simulink model "test_bu01_2018b"  (R2018b)
settings: Solver=FixedStepAuto  StartTime=0.0  StopTime=10  FixedStep=0.02  RelTol=1e-3
model workspace (MAT data in the model file):
  Ixx = 0.8
  Iyy = 2.075
  Izz = 1.25
  K = 0.75
  Mass = 11.5
  b = 0
libraries: simulink x10, aerolibutil x6, vrlib x4, sharedtransform x4, sharedutil x3, shared6dof x1
(part 2 of 4)

== system test_bu01_2018b/bu01_model/动力系统模型/Motor4_TM_N/TMU5KV400  ==
  Um : Inport  PortDimensions=1
  Tq : Inport  Port=2  PortDimensions=1
  Izz : Inport  Port=3  PortDimensions=1
  Bus Selector : BusSelector  OutputSignals=Im,RPM
  Bus Creator : BusCreator  Inputs=3
  DCMotor : Subsystem  mask{L=0.0053, Km=0.024, Kemf=0.024, Imzz=0.00002, Ra=0.113, I0=0.725}
      mask prompts: L "电感值L"; Km "转矩常量Km"; Kemf "反电动势Kemf"; Imzz "转子惯量Imzz"; Ra "电动机内阻Ra"; I0 "空载电流I0"
      mask Display: disp('DCMotor')
  Im : Outport
  RPM : Outport  Port=2
  wires:
  Bus Selector/2 -> RPM/1  "<RPM>"
  Bus Selector/1 -> Im/1  "<Im>"
  DCMotor/1(Out1) -> Bus Selector/1
  Um/1 -> Bus Creator/1  "Um"
  Bus Creator/1 -> DCMotor/1(In1)
  Izz/1 -> Bus Creator/3  "Izz"
  Tq/1 -> Bus Creator/2  "Tq"

== system test_bu01_2018b/bu01_model/动力系统模型/Motor5_PF_N/PF70mmDuctFanN ==
  Vb_ip : Inport  PortDimensions=3
  Wb_ip : Inport  Port=2  PortDimensions=3
  Ax_ip : Inport  Port=3  PortDimensions=3
  Ns_ip : Inport  Port=4  PortDimensions=1
  Pro : Inport  Port=5  PortDimensions=1
  Bus Selector : BusSelector  OutputSignals=Fb&Mb,Tq,Izz
  Bus Selector1 : BusSelector  OutputSignals=Fb,Mb
  Bus Creator : BusCreator  Inputs=5
  "涵道风扇模型 " : Subsystem  mask{Fratio=1.125, Mratio=0.975, Tqratio=0.4, Izz=0.00000309}
      mask prompts: Fratio "涵道风扇气动力修正系数"; Mratio "涵道风扇气动力矩修正系数"; Tqratio "涵道风扇扭矩修正系数"; Izz "涵道风扇转动惯量"
  Fb : Outport
  Mb : Outport  Port=2
  Tq : Outport  Port=3
  Izz : Outport  Port=4
  wires:
  Pro/1 -> Bus Creator/5  "Pro"
  Bus Selector/2 -> Tq/1  "<Tq>"
  Bus Selector/3 -> Izz/1  "<Izz>"
  Bus Selector1/1 -> Fb/1  "<Fb>"
  Ns_ip/1 -> Bus Creator/4  "Ns"
  Bus Selector1/2 -> Mb/1  "<Mb>"
  Bus Selector/1 -> Bus Selector1/1  "<Fb&Mb>"
  Wb_ip/1 -> Bus Creator/2  "Wb"
  Bus Creator/1 -> "涵道风扇模型 "/1(In1)
  "涵道风扇模型 "/1(Out1) -> Bus Selector/1
  Ax_ip/1 -> Bus Creator/3  "Ax"
  Vb_ip/1 -> Bus Creator/1  "Vb"

== system test_bu01_2018b/bu01_model/动力系统模型/Motor5_PF_N/PFKV2300 ==
  Um : Inport  PortDimensions=1
  Tq : Inport  Port=2  PortDimensions=1
  Izz : Inport  Port=3  PortDimensions=1
  Bus Selector : BusSelector  OutputSignals=Im,RPM
  Bus Creator : BusCreator  Inputs=3
  DCMotor : Subsystem  mask{L=0.0053, Km=0.0041, Kemf=0.0041, Imzz=1e-05, Ra=0.045, I0=2.35}
      mask prompts: L "电感值L"; Km "转矩常量Km"; Kemf "反电动势Kemf"; Imzz "转子惯量Imzz"; Ra "电动机内阻Ra"; I0 "空载电流I0"
      mask Display: disp('DCMotor')
  Im : Outport
  RPM : Outport  Port=2
  wires:
  Bus Creator/1 -> DCMotor/1(In1)
  Um/1 -> Bus Creator/1  "Um"
  Izz/1 -> Bus Creator/3  "Izz"
  Bus Selector/2 -> RPM/1  "<RPM>"
  Tq/1 -> Bus Creator/2  "Tq"
  DCMotor/1(Out1) -> Bus Selector/1
  Bus Selector/1 -> Im/1  "<Im>"

== system test_bu01_2018b/bu01_model/动力系统模型/Motor6_PF_N/PF70mmDuctFanN ==
  Vb_ip : Inport  PortDimensions=3
  Wb_ip : Inport  Port=2  PortDimensions=3
  Ax_ip : Inport  Port=3  PortDimensions=3
  Ns_ip : Inport  Port=4  PortDimensions=1
  Pro : Inport  Port=5  PortDimensions=1
  Bus Selector : BusSelector  OutputSignals=Fb&Mb,Tq,Izz
  Bus Selector1 : BusSelector  OutputSignals=Fb,Mb
  Bus Creator : BusCreator  Inputs=5
  "涵道风扇模型 " : Subsystem  mask{Fratio=1.125, Mratio=0.975, Tqratio=0.4, Izz=0.00000309}
      mask prompts: Fratio "涵道风扇气动力修正系数"; Mratio "涵道风扇气动力矩修正系数"; Tqratio "涵道风扇扭矩修正系数"; Izz "涵道风扇转动惯量"
  Fb : Outport
  Mb : Outport  Port=2
  Tq : Outport  Port=3
  Izz : Outport  Port=4
  wires:
  Pro/1 -> Bus Creator/5  "Pro"
  Bus Selector/2 -> Tq/1  "<Tq>"
  Bus Selector/3 -> Izz/1  "<Izz>"
  Bus Selector1/1 -> Fb/1  "<Fb>"
  Ns_ip/1 -> Bus Creator/4  "Ns"
  Bus Selector1/2 -> Mb/1  "<Mb>"
  Bus Selector/1 -> Bus Selector1/1  "<Fb&Mb>"
  Wb_ip/1 -> Bus Creator/2  "Wb"
  Bus Creator/1 -> "涵道风扇模型 "/1(In1)
  "涵道风扇模型 "/1(Out1) -> Bus Selector/1
  Ax_ip/1 -> Bus Creator/3  "Ax"
  Vb_ip/1 -> Bus Creator/1  "Vb"

== system test_bu01_2018b/bu01_model/动力系统模型/Motor6_PF_N/PFKV2300 ==
  Um : Inport  PortDimensions=1
  Tq : Inport  Port=2  PortDimensions=1
  Izz : Inport  Port=3  PortDimensions=1
  Bus Selector : BusSelector  OutputSignals=Im,RPM
  Bus Creator : BusCreator  Inputs=3
  DCMotor : Subsystem  mask{L=0.0053, Km=0.0041, Kemf=0.0041, Imzz=1e-05, Ra=0.045, I0=2.35}
      mask prompts: L "电感值L"; Km "转矩常量Km"; Kemf "反电动势Kemf"; Imzz "转子惯量Imzz"; Ra "电动机内阻Ra"; I0 "空载电流I0"
      mask Display: disp('DCMotor')
  Im : Outport
  RPM : Outport  Port=2
  wires:
  Bus Creator/1 -> DCMotor/1(In1)
  Um/1 -> Bus Creator/1  "Um"
  Izz/1 -> Bus Creator/3  "Izz"
  Bus Selector/2 -> RPM/1  "<RPM>"
  Tq/1 -> Bus Creator/2  "Tq"
  DCMotor/1(Out1) -> Bus Selector/1
  Bus Selector/1 -> Im/1  "<Im>"

== system test_bu01_2018b/bu01_model/动力系统模型/Motor7_PF_N/PF70mmDuctFanN ==
  Vb_ip : Inport  PortDimensions=3
  Wb_ip : Inport  Port=2  PortDimensions=3
  Ax_ip : Inport  Port=3  PortDimensions=3
  Ns_ip : Inport  Port=4  PortDimensions=1
  Pro : Inport  Port=5  PortDimensions=1
  Bus Selector : BusSelector  OutputSignals=Fb&Mb,Tq,Izz
  Bus Selector1 : BusSelector  OutputSignals=Fb,Mb
  Bus Creator : BusCreator  Inputs=5
  "涵道风扇模型 " : Subsystem  mask{Fratio=1.125, Mratio=0.975, Tqratio=0.4, Izz=0.00000309}
      mask prompts: Fratio "涵道风扇气动力修正系数"; Mratio "涵道风扇气动力矩修正系数"; Tqratio "涵道风扇扭矩修正系数"; Izz "涵道风扇转动惯量"
  Fb : Outport
  Mb : Outport  Port=2
  Tq : Outport  Port=3
  Izz : Outport  Port=4
  wires:
  Pro/1 -> Bus Creator/5  "Pro"
  Bus Selector/2 -> Tq/1  "<Tq>"
  Bus Selector/3 -> Izz/1  "<Izz>"
  Bus Selector1/1 -> Fb/1  "<Fb>"
  Ns_ip/1 -> Bus Creator/4  "Ns"
  Bus Selector1/2 -> Mb/1  "<Mb>"
  Bus Selector/1 -> Bus Selector1/1  "<Fb&Mb>"
  Wb_ip/1 -> Bus Creator/2  "Wb"
  Bus Creator/1 -> "涵道风扇模型 "/1(In1)
  "涵道风扇模型 "/1(Out1) -> Bus Selector/1
  Ax_ip/1 -> Bus Creator/3  "Ax"
  Vb_ip/1 -> Bus Creator/1  "Vb"

== system test_bu01_2018b/bu01_model/动力系统模型/Motor7_PF_N/PFKV2300 ==
  Um : Inport  PortDimensions=1
  Tq : Inport  Port=2  PortDimensions=1
  Izz : Inport  Port=3  PortDimensions=1
  Bus Selector : BusSelector  OutputSignals=Im,RPM
  Bus Creator : BusCreator  Inputs=3
  DCMotor : Subsystem  mask{L=0.0053, Km=0.0041, Kemf=0.0041, Imzz=1e-05, Ra=0.045, I0=2.35}
      mask prompts: L "电感值L"; Km "转矩常量Km"; Kemf "反电动势Kemf"; Imzz "转子惯量Imzz"; Ra "电动机内阻Ra"; I0 "空载电流I0"
      mask Display: disp('DCMotor')
  Im : Outport
  RPM : Outport  Port=2
  wires:
  Bus Creator/1 -> DCMotor/1(In1)
  Um/1 -> Bus Creator/1  "Um"
  Izz/1 -> Bus Creator/3  "Izz"
  Bus Selector/2 -> RPM/1  "<RPM>"
  Tq/1 -> Bus Creator/2  "Tq"
  DCMotor/1(Out1) -> Bus Selector/1
  Bus Selector/1 -> Im/1  "<Im>"

== system test_bu01_2018b/bu01_model/动力系统模型/Motor8_PF_N/PF70mmDuctFanN ==
  Vb_ip : Inport  PortDimensions=3
  Wb_ip : Inport  Port=2  PortDimensions=3
  Ax_ip : Inport  Port=3  PortDimensions=3
  Ns_ip : Inport  Port=4  PortDimensions=1
  Pro : Inport  Port=5  PortDimensions=1
  Bus Selector : BusSelector  OutputSignals=Fb&Mb,Tq,Izz
  Bus Selector1 : BusSelector  OutputSignals=Fb,Mb
  Bus Creator : BusCreator  Inputs=5
  "涵道风扇模型 " : Subsystem  mask{Fratio=1.125, Mratio=0.975, Tqratio=0.4, Izz=0.00000309}
      mask prompts: Fratio "涵道风扇气动力修正系数"; Mratio "涵道风扇气动力矩修正系数"; Tqratio "涵道风扇扭矩修正系数"; Izz "涵道风扇转动惯量"
  Fb : Outport
  Mb : Outport  Port=2
  Tq : Outport  Port=3
  Izz : Outport  Port=4
  wires:
  Vb_ip/1 -> Bus Creator/1  "Vb"
  Ax_ip/1 -> Bus Creator/3  "Ax"
  "涵道风扇模型 "/1(Out1) -> Bus Selector/1
  Bus Creator/1 -> "涵道风扇模型 "/1(In1)
  Wb_ip/1 -> Bus Creator/2  "Wb"
  Bus Selector/1 -> Bus Selector1/1  "<Fb&Mb>"
  Bus Selector1/2 -> Mb/1  "<Mb>"
  Ns_ip/1 -> Bus Creator/4  "Ns"
  Bus Selector1/1 -> Fb/1  "<Fb>"
  Bus Selector/3 -> Izz/1  "<Izz>"
  Bus Selector/2 -> Tq/1  "<Tq>"
  Pro/1 -> Bus Creator/5  "Pro"

== system test_bu01_2018b/bu01_model/动力系统模型/Motor8_PF_N/PFKV2300 ==
  Um : Inport  PortDimensions=1
  Tq : Inport  Port=2  PortDimensions=1
  Izz : Inport  Port=3  PortDimensions=1
  Bus Selector : BusSelector  OutputSignals=Im,RPM
  Bus Creator : BusCreator  Inputs=3
  DCMotor : Subsystem  mask{L=0.0053, Km=0.0041, Kemf=0.0041, Imzz=1e-05, Ra=0.045, I0=2.35}
      mask prompts: L "电感值L"; Km "转矩常量Km"; Kemf "反电动势Kemf"; Imzz "转子惯量Imzz"; Ra "电动机内阻Ra"; I0 "空载电流I0"
      mask Display: disp('DCMotor')
  Im : Outport
  RPM : Outport  Port=2
  wires:
  Bus Selector/1 -> Im/1  "<Im>"
  DCMotor/1(Out1) -> Bus Selector/1
  Tq/1 -> Bus Creator/2  "Tq"
  Bus Selector/2 -> RPM/1  "<RPM>"
  Izz/1 -> Bus Creator/3  "Izz"
  Um/1 -> Bus Creator/1  "Um"
  Bus Creator/1 -> DCMotor/1(In1)

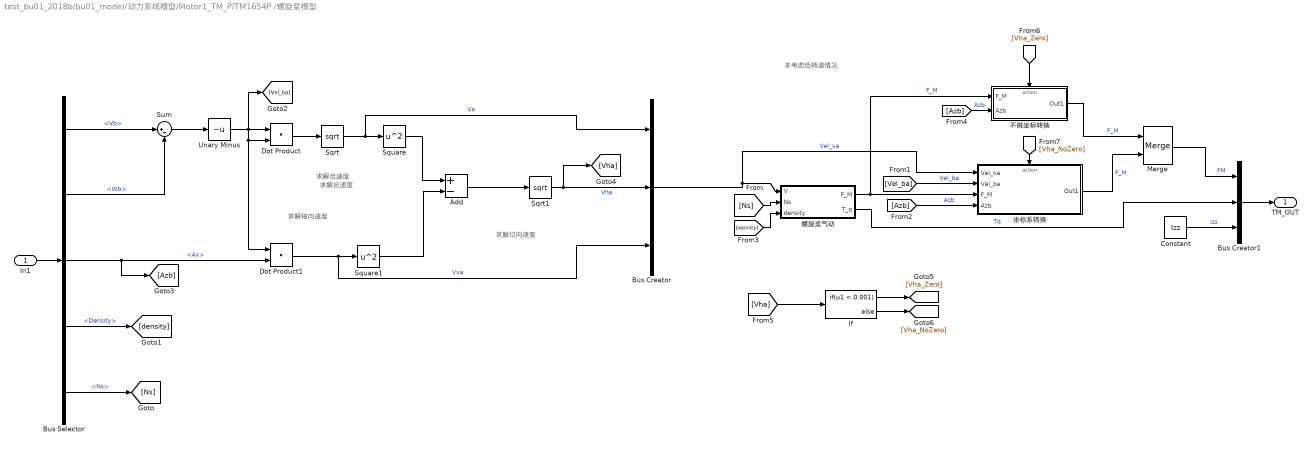
== system test_bu01_2018b/bu01_model/动力系统模型/Motor1_TM_P/TM1654P /螺旋桨模型 ==
  note: 未考虑低转速情况
  note: 求解合速度
  note: 求解轴向速度
  note: 求解切向速度
  note: 求解合速度
  In1 : Inport
  Add : Sum  Inputs=+-
  Bus Selector : BusSelector  OutputSignals=Vb,Wb,Ax,Density,Ns
  Bus Creator : BusCreator  Inputs=3
  Bus Creator1 : BusCreator  Inputs=3
  Constant : Constant  Value=Izz  OutDataTypeStr=double
  Dot Product : DotProduct  InputSameDT=on  OutDataTypeStr=Inherit: Inherit via internal rule
  Dot Product1 : DotProduct  InputSameDT=on  OutDataTypeStr=Inherit: Inherit via internal rule
  If : If  IfExpression=u1 < 0.001
  Merge : Merge
  Sqrt : Sqrt  SaturateOnIntegerOverflow=on
  Sqrt1 : Sqrt  SaturateOnIntegerOverflow=on
  Square : Math  Operator=square  SaturateOnIntegerOverflow=on
  Square1 : Math  Operator=square  SaturateOnIntegerOverflow=on
  Sum : Sum  Inputs=|+-
  Unary Minus : UnaryMinus
  不做坐标转换 : Subsystem
  坐标系转换 : Subsystem
  螺旋桨气动 : Subsystem
  TM_OUT : Outport
  wires:
  In1/1 -> Bus Selector/1
  Bus Selector/1 -> Sum/1  "<Vb>"
  Bus Selector/2 -> Sum/2  "<Wb>"
  Sum/1 -> Unary Minus/1
  Unary Minus/1 -> [Vel_ba], Dot Product/2, Dot Product1/1, Dot Product/1
  Dot Product/1 -> Sqrt/1
  Sqrt/1 -> Bus Creator/1, Square/1  "Va"
  Bus Selector/3 -> [Azb], Dot Product1/2  "<Ax>"
  Bus Selector/4 -> [density]  "<Density>"
  Bus Selector/5 -> [Ns]  "<Ns>"
  Dot Product1/1 -> Bus Creator/3, Square1/1  "Vva"
  Square1/1 -> Add/2
  Square/1 -> Add/1
  Add/1 -> Sqrt1/1
  Sqrt1/1 -> [Vha], Bus Creator/2  "Vha"
  Bus Creator/1 -> 坐标系转换/1(Vel_va), 螺旋桨气动/1(V)  "Vel_va"
  [Ns] -> 螺旋桨气动/2(Ns)
  [Vel_ba] -> 坐标系转换/2(Vel_ba)  "Vel_ba"
  螺旋桨气动/1(F_M) -> 不做坐标转换/1(F_M), 坐标系转换/3(F_M)  "F_M"
  [Azb] -> 坐标系转换/4(Azb)  "Azb"
  [density] -> 螺旋桨气动/3(density)
  螺旋桨气动/2(T_q) -> Bus Creator1/2  "Tq"
  Constant/1 -> Bus Creator1/3  "Izz"
  Bus Creator1/1 -> TM_OUT/1
  [Azb] -> 不做坐标转换/2(Azb)  "Azb"
  [Vha] -> If/1
  不做坐标转换/1(Out1) -> Merge/1  "F_M"
  坐标系转换/1(Out1) -> Merge/2  "F_M"
  Merge/1 -> Bus Creator1/1  "FM"
  If/1 -> [Vha_Zero]
  If/2 -> [Vha_NoZero]
  [Vha_Zero] -> 不做坐标转换/Action
  [Vha_NoZero] -> 坐标系转换/Action

== system test_bu01_2018b/bu01_model/动力系统模型/Motor1_TM_P/TMU5KV400 /DCMotor ==
  In1 : Inport
  Add : Sum  Inputs=+--
  Add1 : Sum  Inputs=+-
  Add2 : Sum
  Add3 : Sum  Inputs=+-
  Bus Selector : BusSelector  OutputSignals=Um,Tq,Izz
  Bus Creator : BusCreator  Inputs=2
  Constant : Constant  Value=Imzz
  Constant1 : Constant  Value=I0
  Divide : Product  Inputs=*/
  Gain : Gain  Gain=1/L
  Gain1 : Gain  Gain=Km
  Gain3 : Gain  Gain=Kemf
  Gain4 : Gain  Gain=Ra
  Gain5 : Gain  Gain=1/(2*pi)
  Gain6 : Gain  Gain=60
  Integrator : Integrator  InitialCondition=0.0001
  Integrator1 : Integrator  InitialCondition=0.0001
  Multiply : Product
  Multiply1 : Product
  Terminator : Terminator
  Terminator1 : Terminator
  Out1 : Outport
  wires:
  In1/1 -> Bus Selector/1
  Bus Selector/1 -> Multiply/1, Add/1  "<Um>"
  Add/1 -> Gain/1
  Gain/1 -> Integrator/1
  Integrator/1 -> Add3/1, Multiply/2, Bus Creator/1, Gain4/1  "Im"
  Gain1/1 -> Multiply1/1, Add1/1  "Te"
  Integrator1/1 -> Multiply1/2, Gain3/1, Gain5/1  "w"
  Add1/1 -> Divide/1
  Divide/1 -> Integrator1/1
  Gain3/1 -> Add/2  "Ea"
  Gain4/1 -> Add/3
  Bus Selector/2 -> [Tq]  "<Tq>"
  Bus Selector/3 -> Add2/1  "<Izz>"
  Constant/1 -> Add2/2
  Add2/1 -> [J]
  [J] -> Divide/2
  Multiply/1 -> Terminator/1  "Pwin"
  Multiply1/1 -> Terminator1/1  "Pwout"
  Gain5/1 -> Gain6/1  "RPS"
  Gain6/1 -> Bus Creator/2  "RPM"
  Bus Creator/1 -> Out1/1
  [Tq] -> Add1/2
  Add3/1 -> Gain1/1  "Iav"
  Constant1/1 -> Add3/2

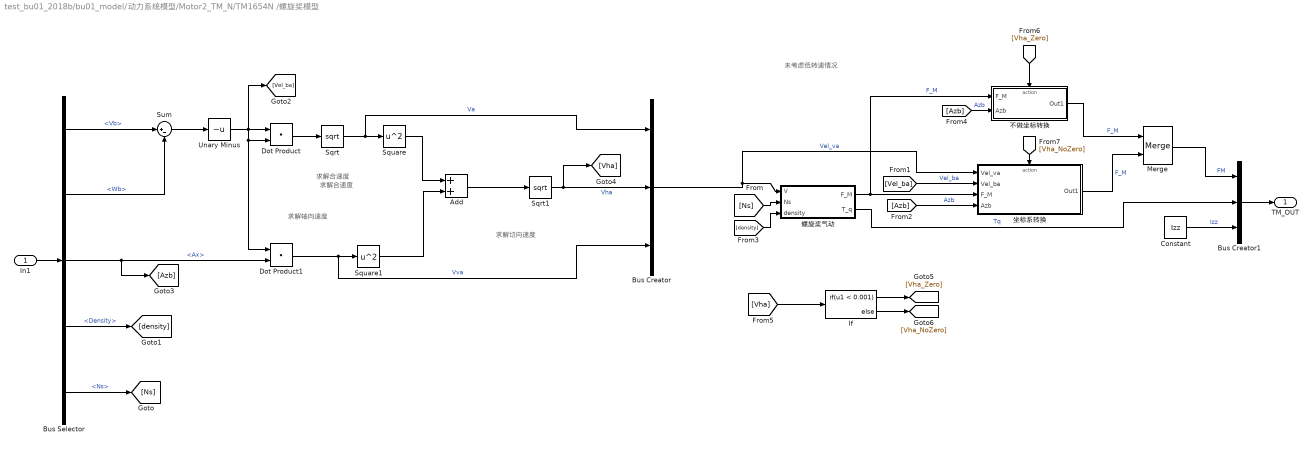
== system test_bu01_2018b/bu01_model/动力系统模型/Motor2_TM_N/TM1654N /螺旋桨模型 ==
  note: 未考虑低转速情况
  note: 求解合速度
  note: 求解轴向速度
  note: 求解切向速度
  note: 求解合速度
  In1 : Inport
  Add : Sum
  Bus Selector : BusSelector  OutputSignals=Vb,Wb,Ax,Density,Ns
  Bus Creator : BusCreator  Inputs=3
  Bus Creator1 : BusCreator  Inputs=3
  Constant : Constant  Value=Izz  OutDataTypeStr=double
  Dot Product : DotProduct  InputSameDT=on  OutDataTypeStr=Inherit: Inherit via internal rule
  Dot Product1 : DotProduct  InputSameDT=on  OutDataTypeStr=Inherit: Inherit via internal rule
  If : If  IfExpression=u1 < 0.001
  Merge : Merge
  Sqrt : Sqrt  SaturateOnIntegerOverflow=on
  Sqrt1 : Sqrt  SaturateOnIntegerOverflow=on
  Square : Math  Operator=square  SaturateOnIntegerOverflow=on
  Square1 : Math  Operator=square  SaturateOnIntegerOverflow=on
  Sum : Sum  Inputs=|+-
  Unary Minus : UnaryMinus
  不做坐标转换 : Subsystem
  坐标系转换 : Subsystem
  螺旋桨气动 : Subsystem
  TM_OUT : Outport
  wires:
  In1/1 -> Bus Selector/1
  Bus Selector/1 -> Sum/1  "<Vb>"
  Bus Selector/2 -> Sum/2  "<Wb>"
  Sum/1 -> Unary Minus/1
  Unary Minus/1 -> [Vel_ba], Dot Product/2, Dot Product1/1, Dot Product/1
  Dot Product/1 -> Sqrt/1
  Sqrt/1 -> Bus Creator/1, Square/1  "Va"
  Bus Selector/3 -> [Azb], Dot Product1/2  "<Ax>"
  Bus Selector/4 -> [density]  "<Density>"
  Bus Selector/5 -> [Ns]  "<Ns>"
  Dot Product1/1 -> Bus Creator/3, Square1/1  "Vva"
  Square1/1 -> Add/2
  Square/1 -> Add/1
  Add/1 -> Sqrt1/1
  Sqrt1/1 -> [Vha], Bus Creator/2  "Vha"
  Bus Creator/1 -> 坐标系转换/1(Vel_va), 螺旋桨气动/1(V)  "Vel_va"
  [Ns] -> 螺旋桨气动/2(Ns)
  [Vel_ba] -> 坐标系转换/2(Vel_ba)  "Vel_ba"
  螺旋桨气动/1(F_M) -> 不做坐标转换/1(F_M), 坐标系转换/3(F_M)  "F_M"
  [Azb] -> 坐标系转换/4(Azb)  "Azb"
  [density] -> 螺旋桨气动/3(density)
  螺旋桨气动/2(T_q) -> Bus Creator1/2  "Tq"
  Constant/1 -> Bus Creator1/3  "Izz"
  Bus Creator1/1 -> TM_OUT/1
  [Azb] -> 不做坐标转换/2(Azb)  "Azb"
  [Vha] -> If/1
  不做坐标转换/1(Out1) -> Merge/1  "F_M"
  坐标系转换/1(Out1) -> Merge/2  "F_M"
  Merge/1 -> Bus Creator1/1  "FM"
  If/1 -> [Vha_Zero]
  If/2 -> [Vha_NoZero]
  [Vha_Zero] -> 不做坐标转换/Action
  [Vha_NoZero] -> 坐标系转换/Action

== system test_bu01_2018b/bu01_model/动力系统模型/Motor2_TM_N/TMU5KV400 /DCMotor ==
  In1 : Inport
  Add : Sum  Inputs=+--
  Add1 : Sum  Inputs=+-
  Add2 : Sum
  Add3 : Sum  Inputs=+-
  Bus Selector : BusSelector  OutputSignals=Um,Tq,Izz
  Bus Creator : BusCreator  Inputs=2
  Constant : Constant  Value=Imzz
  Constant1 : Constant  Value=I0
  Divide : Product  Inputs=*/
  Gain : Gain  Gain=1/L
  Gain1 : Gain  Gain=Km
  Gain3 : Gain  Gain=Kemf
  Gain4 : Gain  Gain=Ra
  Gain5 : Gain  Gain=1/(2*pi)
  Gain6 : Gain  Gain=60
  Integrator : Integrator  InitialCondition=0.0001
  Integrator1 : Integrator  InitialCondition=0.0001
  Multiply : Product
  Multiply1 : Product
  Terminator : Terminator
  Terminator1 : Terminator
  Out1 : Outport
  wires:
  In1/1 -> Bus Selector/1
  Bus Selector/1 -> Multiply/1, Add/1  "<Um>"
  Add/1 -> Gain/1
  Gain/1 -> Integrator/1
  Integrator/1 -> Add3/1, Multiply/2, Bus Creator/1, Gain4/1  "Im"
  Gain1/1 -> Multiply1/1, Add1/1  "Te"
  Integrator1/1 -> Multiply1/2, Gain3/1, Gain5/1  "w"
  Add1/1 -> Divide/1
  Divide/1 -> Integrator1/1
  Gain3/1 -> Add/2  "Ea"
  Gain4/1 -> Add/3
  Bus Selector/2 -> [Tq]  "<Tq>"
  Bus Selector/3 -> Add2/1  "<Izz>"
  Constant/1 -> Add2/2
  Add2/1 -> [J]
  [J] -> Divide/2
  Multiply/1 -> Terminator/1  "Pwin"
  Multiply1/1 -> Terminator1/1  "Pwout"
  Gain5/1 -> Gain6/1  "RPS"
  Gain6/1 -> Bus Creator/2  "RPM"
  Bus Creator/1 -> Out1/1
  [Tq] -> Add1/2
  Add3/1 -> Gain1/1  "Iav"
  Constant1/1 -> Add3/2

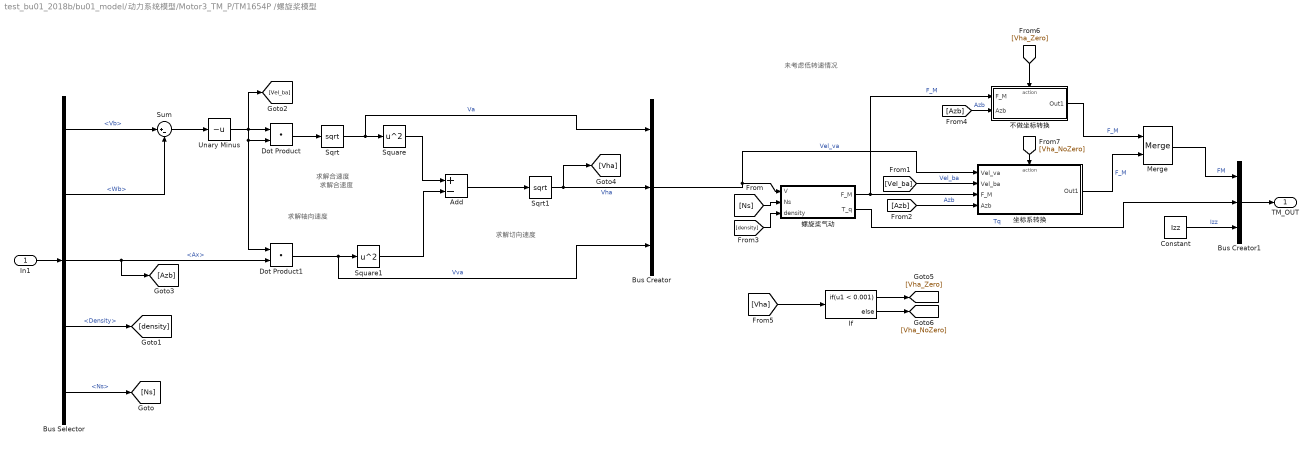
== system test_bu01_2018b/bu01_model/动力系统模型/Motor3_TM_P/TM1654P /螺旋桨模型 ==
  note: 未考虑低转速情况
  note: 求解合速度
  note: 求解轴向速度
  note: 求解切向速度
  note: 求解合速度
  In1 : Inport
  Add : Sum  Inputs=+-
  Bus Selector : BusSelector  OutputSignals=Vb,Wb,Ax,Density,Ns
  Bus Creator : BusCreator  Inputs=3
  Bus Creator1 : BusCreator  Inputs=3
  Constant : Constant  Value=Izz  OutDataTypeStr=double
  Dot Product : DotProduct  InputSameDT=on  OutDataTypeStr=Inherit: Inherit via internal rule
  Dot Product1 : DotProduct  InputSameDT=on  OutDataTypeStr=Inherit: Inherit via internal rule
  If : If  IfExpression=u1 < 0.001
  Merge : Merge
  Sqrt : Sqrt  SaturateOnIntegerOverflow=on
  Sqrt1 : Sqrt  SaturateOnIntegerOverflow=on
  Square : Math  Operator=square  SaturateOnIntegerOverflow=on
  Square1 : Math  Operator=square  SaturateOnIntegerOverflow=on
  Sum : Sum  Inputs=|+-
  Unary Minus : UnaryMinus
  不做坐标转换 : Subsystem
  坐标系转换 : Subsystem
  螺旋桨气动 : Subsystem
  TM_OUT : Outport
  wires:
  In1/1 -> Bus Selector/1
  Bus Selector/1 -> Sum/1  "<Vb>"
  Bus Selector/2 -> Sum/2  "<Wb>"
  Sum/1 -> Unary Minus/1
  Unary Minus/1 -> [Vel_ba], Dot Product/2, Dot Product1/1, Dot Product/1
  Dot Product/1 -> Sqrt/1
  Sqrt/1 -> Bus Creator/1, Square/1  "Va"
  Bus Selector/3 -> [Azb], Dot Product1/2  "<Ax>"
  Bus Selector/4 -> [density]  "<Density>"
  Bus Selector/5 -> [Ns]  "<Ns>"
  Dot Product1/1 -> Bus Creator/3, Square1/1  "Vva"
  Square1/1 -> Add/2
  Square/1 -> Add/1
  Add/1 -> Sqrt1/1
  Sqrt1/1 -> [Vha], Bus Creator/2  "Vha"
  Bus Creator/1 -> 坐标系转换/1(Vel_va), 螺旋桨气动/1(V)  "Vel_va"
  [Ns] -> 螺旋桨气动/2(Ns)
  [Vel_ba] -> 坐标系转换/2(Vel_ba)  "Vel_ba"
  螺旋桨气动/1(F_M) -> 不做坐标转换/1(F_M), 坐标系转换/3(F_M)  "F_M"
  [Azb] -> 坐标系转换/4(Azb)  "Azb"
  [density] -> 螺旋桨气动/3(density)
  螺旋桨气动/2(T_q) -> Bus Creator1/2  "Tq"
  Constant/1 -> Bus Creator1/3  "Izz"
  Bus Creator1/1 -> TM_OUT/1
  [Azb] -> 不做坐标转换/2(Azb)  "Azb"
  [Vha] -> If/1
  不做坐标转换/1(Out1) -> Merge/1  "F_M"
  坐标系转换/1(Out1) -> Merge/2  "F_M"
  Merge/1 -> Bus Creator1/1  "FM"
  If/1 -> [Vha_Zero]
  If/2 -> [Vha_NoZero]
  [Vha_Zero] -> 不做坐标转换/Action
  [Vha_NoZero] -> 坐标系转换/Action

== system test_bu01_2018b/bu01_model/动力系统模型/Motor3_TM_P/TMU5KV400 /DCMotor ==
  In1 : Inport
  Add : Sum  Inputs=+--
  Add1 : Sum  Inputs=+-
  Add2 : Sum
  Add3 : Sum  Inputs=+-
  Bus Selector : BusSelector  OutputSignals=Um,Tq,Izz
  Bus Creator : BusCreator  Inputs=2
  Constant : Constant  Value=Imzz
  Constant1 : Constant  Value=I0
  Divide : Product  Inputs=*/
  Gain : Gain  Gain=1/L
  Gain1 : Gain  Gain=Km
  Gain3 : Gain  Gain=Kemf
  Gain4 : Gain  Gain=Ra
  Gain5 : Gain  Gain=1/(2*pi)
  Gain6 : Gain  Gain=60
  Integrator : Integrator  InitialCondition=0.0001
  Integrator1 : Integrator  InitialCondition=0.0001
  Multiply : Product
  Multiply1 : Product
  Terminator : Terminator
  Terminator1 : Terminator
  Out1 : Outport
  wires:
  In1/1 -> Bus Selector/1
  Bus Selector/1 -> Multiply/1, Add/1  "<Um>"
  Add/1 -> Gain/1
  Gain/1 -> Integrator/1
  Integrator/1 -> Add3/1, Multiply/2, Bus Creator/1, Gain4/1  "Im"
  Gain1/1 -> Multiply1/1, Add1/1  "Te"
  Integrator1/1 -> Multiply1/2, Gain3/1, Gain5/1  "w"
  Add1/1 -> Divide/1
  Divide/1 -> Integrator1/1
  Gain3/1 -> Add/2  "Ea"
  Gain4/1 -> Add/3
  Bus Selector/2 -> [Tq]  "<Tq>"
  Bus Selector/3 -> Add2/1  "<Izz>"
  Constant/1 -> Add2/2
  Add2/1 -> [J]
  [J] -> Divide/2
  Multiply/1 -> Terminator/1  "Pwin"
  Multiply1/1 -> Terminator1/1  "Pwout"
  Gain5/1 -> Gain6/1  "RPS"
  Gain6/1 -> Bus Creator/2  "RPM"
  Bus Creator/1 -> Out1/1
  [Tq] -> Add1/2
  Add3/1 -> Gain1/1  "Iav"
  Constant1/1 -> Add3/2

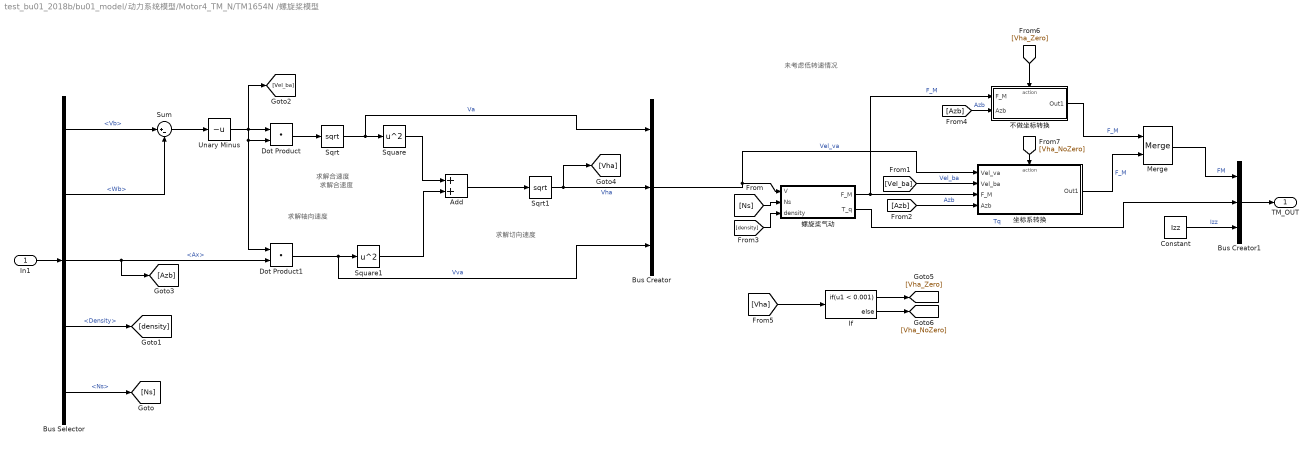
== system test_bu01_2018b/bu01_model/动力系统模型/Motor4_TM_N/TM1654N /螺旋桨模型 ==
  note: 未考虑低转速情况
  note: 求解合速度
  note: 求解轴向速度
  note: 求解切向速度
  note: 求解合速度
  In1 : Inport
  Add : Sum
  Bus Selector : BusSelector  OutputSignals=Vb,Wb,Ax,Density,Ns
  Bus Creator : BusCreator  Inputs=3
  Bus Creator1 : BusCreator  Inputs=3
  Constant : Constant  Value=Izz  OutDataTypeStr=double
  Dot Product : DotProduct  InputSameDT=on  OutDataTypeStr=Inherit: Inherit via internal rule
  Dot Product1 : DotProduct  InputSameDT=on  OutDataTypeStr=Inherit: Inherit via internal rule
  If : If  IfExpression=u1 < 0.001
  Merge : Merge
  Sqrt : Sqrt  SaturateOnIntegerOverflow=on
  Sqrt1 : Sqrt  SaturateOnIntegerOverflow=on
  Square : Math  Operator=square  SaturateOnIntegerOverflow=on
  Square1 : Math  Operator=square  SaturateOnIntegerOverflow=on
  Sum : Sum  Inputs=|+-
  Unary Minus : UnaryMinus
  不做坐标转换 : Subsystem
  坐标系转换 : Subsystem
  螺旋桨气动 : Subsystem
  TM_OUT : Outport
  wires:
  In1/1 -> Bus Selector/1
  Bus Selector/1 -> Sum/1  "<Vb>"
  Bus Selector/2 -> Sum/2  "<Wb>"
  Sum/1 -> Unary Minus/1
  Unary Minus/1 -> [Vel_ba], Dot Product/2, Dot Product1/1, Dot Product/1
  Dot Product/1 -> Sqrt/1
  Sqrt/1 -> Bus Creator/1, Square/1  "Va"
  Bus Selector/3 -> [Azb], Dot Product1/2  "<Ax>"
  Bus Selector/4 -> [density]  "<Density>"
  Bus Selector/5 -> [Ns]  "<Ns>"
  Dot Product1/1 -> Bus Creator/3, Square1/1  "Vva"
  Square1/1 -> Add/2
  Square/1 -> Add/1
  Add/1 -> Sqrt1/1
  Sqrt1/1 -> [Vha], Bus Creator/2  "Vha"
  Bus Creator/1 -> 坐标系转换/1(Vel_va), 螺旋桨气动/1(V)  "Vel_va"
  [Ns] -> 螺旋桨气动/2(Ns)
  [Vel_ba] -> 坐标系转换/2(Vel_ba)  "Vel_ba"
  螺旋桨气动/1(F_M) -> 不做坐标转换/1(F_M), 坐标系转换/3(F_M)  "F_M"
  [Azb] -> 坐标系转换/4(Azb)  "Azb"
  [density] -> 螺旋桨气动/3(density)
  螺旋桨气动/2(T_q) -> Bus Creator1/2  "Tq"
  Constant/1 -> Bus Creator1/3  "Izz"
  Bus Creator1/1 -> TM_OUT/1
  [Azb] -> 不做坐标转换/2(Azb)  "Azb"
  [Vha] -> If/1
  不做坐标转换/1(Out1) -> Merge/1  "F_M"
  坐标系转换/1(Out1) -> Merge/2  "F_M"
  Merge/1 -> Bus Creator1/1  "FM"
  If/1 -> [Vha_Zero]
  If/2 -> [Vha_NoZero]
  [Vha_Zero] -> 不做坐标转换/Action
  [Vha_NoZero] -> 坐标系转换/Action

== system test_bu01_2018b/bu01_model/动力系统模型/Motor4_TM_N/TMU5KV400 /DCMotor ==
  In1 : Inport
  Add : Sum  Inputs=+--
  Add1 : Sum  Inputs=+-
  Add2 : Sum
  Add3 : Sum  Inputs=+-
  Bus Selector : BusSelector  OutputSignals=Um,Tq,Izz
  Bus Creator : BusCreator  Inputs=2
  Constant : Constant  Value=Imzz
  Constant1 : Constant  Value=I0
  Divide : Product  Inputs=*/
  Gain : Gain  Gain=1/L
  Gain1 : Gain  Gain=Km
  Gain3 : Gain  Gain=Kemf
  Gain4 : Gain  Gain=Ra
  Gain5 : Gain  Gain=1/(2*pi)
  Gain6 : Gain  Gain=60
  Integrator : Integrator  InitialCondition=0.0001
  Integrator1 : Integrator  InitialCondition=0.0001
  Multiply : Product
  Multiply1 : Product
  Terminator : Terminator
  Terminator1 : Terminator
  Out1 : Outport
  wires:
  In1/1 -> Bus Selector/1
  Bus Selector/1 -> Multiply/1, Add/1  "<Um>"
  Add/1 -> Gain/1
  Gain/1 -> Integrator/1
  Integrator/1 -> Add3/1, Multiply/2, Bus Creator/1, Gain4/1  "Im"
  Gain1/1 -> Multiply1/1, Add1/1  "Te"
  Integrator1/1 -> Multiply1/2, Gain3/1, Gain5/1  "w"
  Add1/1 -> Divide/1
  Divide/1 -> Integrator1/1
  Gain3/1 -> Add/2  "Ea"
  Gain4/1 -> Add/3
  Bus Selector/2 -> [Tq]  "<Tq>"
  Bus Selector/3 -> Add2/1  "<Izz>"
  Constant/1 -> Add2/2
  Add2/1 -> [J]
  [J] -> Divide/2
  Multiply/1 -> Terminator/1  "Pwin"
  Multiply1/1 -> Terminator1/1  "Pwout"
  Gain5/1 -> Gain6/1  "RPS"
  Gain6/1 -> Bus Creator/2  "RPM"
  Bus Creator/1 -> Out1/1
  [Tq] -> Add1/2
  Add3/1 -> Gain1/1  "Iav"
  Constant1/1 -> Add3/2

== system test_bu01_2018b/bu01_model/动力系统模型/Motor5_PF_N/PF70mmDuctFanN/涵道风扇模型  ==
  In1 : Inport
  Bus Creator : BusCreator  Inputs=7
  Bus Selector : BusSelector  OutputSignals=Vb,Wb,Ax,Ns,Pro
  If : If  IfExpression=u1 > 1
  Merge : Merge
  Sum : Sum  Inputs=|+-
  Sum1 : Sum  Inputs=|+-
  Terminator : Terminator
  Va : Sqrt  SaturateOnIntegerOverflow=on
  Va^2 : DotProduct  InputSameDT=on  OutDataTypeStr=Inherit: Inherit via internal rule
  Vha : Sqrt  SaturateOnIntegerOverflow=on
  Vva : DotProduct  InputSameDT=on  OutDataTypeStr=Inherit: Inherit via internal rule
  Vva1 : UnaryMinus
  Vva^2 : Math  Operator=square  SaturateOnIntegerOverflow=on
  "[Uba,Vba,Wba]" : UnaryMinus
  求解涵道风扇气动载荷 : Subsystem  TreatAsAtomicUnit=on
  转速太低无载荷输出 : Subsystem  TreatAsAtomicUnit=on
  Out1 : Outport
  wires:
  Bus Selector/1 -> Sum/1  "<Vb>"
  In1/1 -> Bus Selector/1
  Bus Selector/2 -> Sum/2  "<Wb>"
  Sum/1 -> "[Uba,Vba,Wba]"/1
  "[Uba,Vba,Wba]"/1 -> Bus Creator/1, Vva/1, Va^2/2, Va^2/1  "Vba"
  Bus Selector/3 -> Bus Creator/4, Vva/2  "<Ax>"
  Va^2/1 -> Sum1/1, Va/1
  Vva/1 -> Bus Creator/7, Vva^2/1, Vva1/1  "Vva"
  Vva^2/1 -> Sum1/2
  Sum1/1 -> Vha/1
  Vha/1 -> Bus Creator/2  "Vha"
  Vva1/1 -> Bus Creator/3  "Vva1"
  Bus Selector/4 -> Bus Creator/5, If/1  "<Ns>"
  If/1 -> 求解涵道风扇气动载荷/Action
  If/2 -> 转速太低无载荷输出/Action
  Bus Selector/5 -> Bus Creator/6  "<Pro>"
  Bus Creator/1 -> 求解涵道风扇气动载荷/1(In1)
  求解涵道风扇气动载荷/1(Out1) -> Merge/1  "Fb&Mb"
  转速太低无载荷输出/1(Out1) -> Merge/2  "Fb&Mb"
  Va/1 -> Terminator/1  "Va"
  Merge/1 -> Out1/1  "Fb&Mb"

== system test_bu01_2018b/bu01_model/动力系统模型/Motor5_PF_N/PFKV2300/DCMotor ==
  In1 : Inport
  Add : Sum  Inputs=+--
  Add1 : Sum  Inputs=+-
  Add2 : Sum
  Add3 : Sum  Inputs=+-
  Bus Selector : BusSelector  OutputSignals=Um,Tq,Izz
  Bus Creator : BusCreator  Inputs=2
  Constant : Constant  Value=Imzz
  Constant1 : Constant  Value=I0
  Divide : Product  Inputs=*/
  Gain : Gain  Gain=1/L
  Gain1 : Gain  Gain=Km
  Gain3 : Gain  Gain=Kemf
  Gain4 : Gain  Gain=Ra
  Gain5 : Gain  Gain=1/(2*pi)
  Gain6 : Gain  Gain=60
  Integrator : Integrator
  Integrator1 : Integrator
  Multiply : Product
  Multiply1 : Product
  Terminator : Terminator
  Terminator1 : Terminator
  Out1 : Outport
  wires:
  In1/1 -> Bus Selector/1
  Bus Selector/1 -> Multiply/1, Add/1  "<Um>"
  Add/1 -> Gain/1
  Gain/1 -> Integrator/1
  Integrator/1 -> Add3/1, Multiply/2, Bus Creator/1, Gain4/1  "Im"
  Gain1/1 -> Multiply1/1, Add1/1  "Te"
  Integrator1/1 -> Multiply1/2, Gain3/1, Gain5/1  "w"
  Add1/1 -> Divide/1
  Divide/1 -> Integrator1/1
  Gain3/1 -> Add/2  "Ea"
  Gain4/1 -> Add/3
  Bus Selector/2 -> [Tq]  "<Tq>"
  Bus Selector/3 -> Add2/1  "<Izz>"
  Constant/1 -> Add2/2
  Add2/1 -> [J]
  [J] -> Divide/2
  Multiply/1 -> Terminator/1  "Pwin"
  Multiply1/1 -> Terminator1/1  "Pwout"
  Gain5/1 -> Gain6/1  "RPS"
  Gain6/1 -> Bus Creator/2  "RPM"
  Bus Creator/1 -> Out1/1
  [Tq] -> Add1/2
  Add3/1 -> Gain1/1  "Iav"
  Constant1/1 -> Add3/2

== system test_bu01_2018b/bu01_model/动力系统模型/Motor6_PF_N/PF70mmDuctFanN/涵道风扇模型  ==
  In1 : Inport
  Bus Creator : BusCreator  Inputs=7
  Bus Selector : BusSelector  OutputSignals=Vb,Wb,Ax,Ns,Pro
  If : If  IfExpression=u1 > 1
  Merge : Merge
  Sum : Sum  Inputs=|+-
  Sum1 : Sum  Inputs=|+-
  Terminator : Terminator
  Va : Sqrt  SaturateOnIntegerOverflow=on
  Va^2 : DotProduct  InputSameDT=on  OutDataTypeStr=Inherit: Inherit via internal rule
  Vha : Sqrt  SaturateOnIntegerOverflow=on
  Vva : DotProduct  InputSameDT=on  OutDataTypeStr=Inherit: Inherit via internal rule
  Vva1 : UnaryMinus
  Vva^2 : Math  Operator=square  SaturateOnIntegerOverflow=on
  "[Uba,Vba,Wba]" : UnaryMinus
  求解涵道风扇气动载荷 : Subsystem  TreatAsAtomicUnit=on
  转速太低无载荷输出 : Subsystem  TreatAsAtomicUnit=on
  Out1 : Outport
  wires:
  Bus Selector/1 -> Sum/1  "<Vb>"
  In1/1 -> Bus Selector/1
  Bus Selector/2 -> Sum/2  "<Wb>"
  Sum/1 -> "[Uba,Vba,Wba]"/1
  "[Uba,Vba,Wba]"/1 -> Bus Creator/1, Vva/1, Va^2/2, Va^2/1  "Vba"
  Bus Selector/3 -> Bus Creator/4, Vva/2  "<Ax>"
  Va^2/1 -> Sum1/1, Va/1
  Vva/1 -> Bus Creator/7, Vva^2/1, Vva1/1  "Vva"
  Vva^2/1 -> Sum1/2
  Sum1/1 -> Vha/1
  Vha/1 -> Bus Creator/2  "Vha"
  Vva1/1 -> Bus Creator/3  "Vva1"
  Bus Selector/4 -> Bus Creator/5, If/1  "<Ns>"
  If/1 -> 求解涵道风扇气动载荷/Action
  If/2 -> 转速太低无载荷输出/Action
  Bus Selector/5 -> Bus Creator/6  "<Pro>"
  Bus Creator/1 -> 求解涵道风扇气动载荷/1(In1)
  求解涵道风扇气动载荷/1(Out1) -> Merge/1  "Fb&Mb"
  转速太低无载荷输出/1(Out1) -> Merge/2  "Fb&Mb"
  Va/1 -> Terminator/1  "Va"
  Merge/1 -> Out1/1  "Fb&Mb"

== system test_bu01_2018b/bu01_model/动力系统模型/Motor6_PF_N/PFKV2300/DCMotor ==
  In1 : Inport
  Add : Sum  Inputs=+--
  Add1 : Sum  Inputs=+-
  Add2 : Sum
  Add3 : Sum  Inputs=+-
  Bus Selector : BusSelector  OutputSignals=Um,Tq,Izz
  Bus Creator : BusCreator  Inputs=2
  Constant : Constant  Value=Imzz
  Constant1 : Constant  Value=I0
  Divide : Product  Inputs=*/
  Gain : Gain  Gain=1/L
  Gain1 : Gain  Gain=Km
  Gain3 : Gain  Gain=Kemf
  Gain4 : Gain  Gain=Ra
  Gain5 : Gain  Gain=1/(2*pi)
  Gain6 : Gain  Gain=60
  Integrator : Integrator
  Integrator1 : Integrator
  Multiply : Product
  Multiply1 : Product
  Terminator : Terminator
  Terminator1 : Terminator
  Out1 : Outport
  wires:
  In1/1 -> Bus Selector/1
  Bus Selector/1 -> Multiply/1, Add/1  "<Um>"
  Add/1 -> Gain/1
  Gain/1 -> Integrator/1
  Integrator/1 -> Add3/1, Multiply/2, Bus Creator/1, Gain4/1  "Im"
  Gain1/1 -> Multiply1/1, Add1/1  "Te"
  Integrator1/1 -> Multiply1/2, Gain3/1, Gain5/1  "w"
  Add1/1 -> Divide/1
  Divide/1 -> Integrator1/1
  Gain3/1 -> Add/2  "Ea"
  Gain4/1 -> Add/3
  Bus Selector/2 -> [Tq]  "<Tq>"
  Bus Selector/3 -> Add2/1  "<Izz>"
  Constant/1 -> Add2/2
  Add2/1 -> [J]
  [J] -> Divide/2
  Multiply/1 -> Terminator/1  "Pwin"
  Multiply1/1 -> Terminator1/1  "Pwout"
  Gain5/1 -> Gain6/1  "RPS"
  Gain6/1 -> Bus Creator/2  "RPM"
  Bus Creator/1 -> Out1/1
  [Tq] -> Add1/2
  Add3/1 -> Gain1/1  "Iav"
  Constant1/1 -> Add3/2

== system test_bu01_2018b/bu01_model/动力系统模型/Motor7_PF_N/PF70mmDuctFanN/涵道风扇模型  ==
  In1 : Inport
  Bus Creator : BusCreator  Inputs=7
  Bus Selector : BusSelector  OutputSignals=Vb,Wb,Ax,Ns,Pro
  If : If  IfExpression=u1 > 1
  Merge : Merge
  Sum : Sum  Inputs=|+-
  Sum1 : Sum  Inputs=|+-
  Terminator : Terminator
  Va : Sqrt  SaturateOnIntegerOverflow=on
  Va^2 : DotProduct  InputSameDT=on  OutDataTypeStr=Inherit: Inherit via internal rule
  Vha : Sqrt  SaturateOnIntegerOverflow=on
  Vva : DotProduct  InputSameDT=on  OutDataTypeStr=Inherit: Inherit via internal rule
  Vva1 : UnaryMinus
  Vva^2 : Math  Operator=square  SaturateOnIntegerOverflow=on
  "[Uba,Vba,Wba]" : UnaryMinus
  求解涵道风扇气动载荷 : Subsystem  TreatAsAtomicUnit=on
  转速太低无载荷输出 : Subsystem  TreatAsAtomicUnit=on
  Out1 : Outport
  wires:
  Bus Selector/1 -> Sum/1  "<Vb>"
  In1/1 -> Bus Selector/1
  Bus Selector/2 -> Sum/2  "<Wb>"
  Sum/1 -> "[Uba,Vba,Wba]"/1
  "[Uba,Vba,Wba]"/1 -> Bus Creator/1, Vva/1, Va^2/2, Va^2/1  "Vba"
  Bus Selector/3 -> Bus Creator/4, Vva/2  "<Ax>"
  Va^2/1 -> Sum1/1, Va/1
  Vva/1 -> Bus Creator/7, Vva^2/1, Vva1/1  "Vva"
  Vva^2/1 -> Sum1/2
  Sum1/1 -> Vha/1
  Vha/1 -> Bus Creator/2  "Vha"
  Vva1/1 -> Bus Creator/3  "Vva1"
  Bus Selector/4 -> Bus Creator/5, If/1  "<Ns>"
  If/1 -> 求解涵道风扇气动载荷/Action
  If/2 -> 转速太低无载荷输出/Action
  Bus Selector/5 -> Bus Creator/6  "<Pro>"
  Bus Creator/1 -> 求解涵道风扇气动载荷/1(In1)
  求解涵道风扇气动载荷/1(Out1) -> Merge/1  "Fb&Mb"
  转速太低无载荷输出/1(Out1) -> Merge/2  "Fb&Mb"
  Va/1 -> Terminator/1  "Va"
  Merge/1 -> Out1/1  "Fb&Mb"

== system test_bu01_2018b/bu01_model/动力系统模型/Motor7_PF_N/PFKV2300/DCMotor ==
  In1 : Inport
  Add : Sum  Inputs=+--
  Add1 : Sum  Inputs=+-
  Add2 : Sum
  Add3 : Sum  Inputs=+-
  Bus Selector : BusSelector  OutputSignals=Um,Tq,Izz
  Bus Creator : BusCreator  Inputs=2
  Constant : Constant  Value=Imzz
  Constant1 : Constant  Value=I0
  Divide : Product  Inputs=*/
  Gain : Gain  Gain=1/L
  Gain1 : Gain  Gain=Km
  Gain3 : Gain  Gain=Kemf
  Gain4 : Gain  Gain=Ra
  Gain5 : Gain  Gain=1/(2*pi)
  Gain6 : Gain  Gain=60
  Integrator : Integrator
  Integrator1 : Integrator
  Multiply : Product
  Multiply1 : Product
  Terminator : Terminator
  Terminator1 : Terminator
  Out1 : Outport
  wires:
  In1/1 -> Bus Selector/1
  Bus Selector/1 -> Multiply/1, Add/1  "<Um>"
  Add/1 -> Gain/1
  Gain/1 -> Integrator/1
  Integrator/1 -> Add3/1, Multiply/2, Bus Creator/1, Gain4/1  "Im"
  Gain1/1 -> Multiply1/1, Add1/1  "Te"
  Integrator1/1 -> Multiply1/2, Gain3/1, Gain5/1  "w"
  Add1/1 -> Divide/1
  Divide/1 -> Integrator1/1
  Gain3/1 -> Add/2  "Ea"
  Gain4/1 -> Add/3
  Bus Selector/2 -> [Tq]  "<Tq>"
  Bus Selector/3 -> Add2/1  "<Izz>"
  Constant/1 -> Add2/2
  Add2/1 -> [J]
  [J] -> Divide/2
  Multiply/1 -> Terminator/1  "Pwin"
  Multiply1/1 -> Terminator1/1  "Pwout"
  Gain5/1 -> Gain6/1  "RPS"
  Gain6/1 -> Bus Creator/2  "RPM"
  Bus Creator/1 -> Out1/1
  [Tq] -> Add1/2
  Add3/1 -> Gain1/1  "Iav"
  Constant1/1 -> Add3/2

== system test_bu01_2018b/bu01_model/动力系统模型/Motor8_PF_N/PF70mmDuctFanN/涵道风扇模型  ==
  In1 : Inport
  Bus Creator : BusCreator  Inputs=7
  Bus Selector : BusSelector  OutputSignals=Vb,Wb,Ax,Ns,Pro
  If : If  IfExpression=u1 > 1
  Merge : Merge
  Sum : Sum  Inputs=|+-
  Sum1 : Sum  Inputs=|+-
  Terminator : Terminator
  Va : Sqrt  SaturateOnIntegerOverflow=on
  Va^2 : DotProduct  InputSameDT=on  OutDataTypeStr=Inherit: Inherit via internal rule
  Vha : Sqrt  SaturateOnIntegerOverflow=on
  Vva : DotProduct  InputSameDT=on  OutDataTypeStr=Inherit: Inherit via internal rule
  Vva1 : UnaryMinus
  Vva^2 : Math  Operator=square  SaturateOnIntegerOverflow=on
  "[Uba,Vba,Wba]" : UnaryMinus
  求解涵道风扇气动载荷 : Subsystem  TreatAsAtomicUnit=on
  转速太低无载荷输出 : Subsystem  TreatAsAtomicUnit=on
  Out1 : Outport
  wires:
  Merge/1 -> Out1/1  "Fb&Mb"
  Va/1 -> Terminator/1  "Va"
  转速太低无载荷输出/1(Out1) -> Merge/2  "Fb&Mb"
  求解涵道风扇气动载荷/1(Out1) -> Merge/1  "Fb&Mb"
  Bus Creator/1 -> 求解涵道风扇气动载荷/1(In1)
  Bus Selector/5 -> Bus Creator/6  "<Pro>"
  If/2 -> 转速太低无载荷输出/Action
  If/1 -> 求解涵道风扇气动载荷/Action
  Bus Selector/4 -> If/1, Bus Creator/5  "<Ns>"
  Vva1/1 -> Bus Creator/3  "Vva1"
  Vha/1 -> Bus Creator/2  "Vha"
  Sum1/1 -> Vha/1
  Vva^2/1 -> Sum1/2
  Vva/1 -> Vva1/1, Vva^2/1, Bus Creator/7  "Vva"
  Va^2/1 -> Va/1, Sum1/1
  Bus Selector/3 -> Vva/2, Bus Creator/4  "<Ax>"
  "[Uba,Vba,Wba]"/1 -> Va^2/1, Va^2/2, Vva/1, Bus Creator/1  "Vba"
  Sum/1 -> "[Uba,Vba,Wba]"/1
  Bus Selector/2 -> Sum/2  "<Wb>"
  In1/1 -> Bus Selector/1
  Bus Selector/1 -> Sum/1  "<Vb>"

== system test_bu01_2018b/bu01_model/动力系统模型/Motor8_PF_N/PFKV2300/DCMotor ==
  In1 : Inport
  Add : Sum  Inputs=+--
  Add1 : Sum  Inputs=+-
  Add2 : Sum
  Add3 : Sum  Inputs=+-
  Bus Selector : BusSelector  OutputSignals=Um,Tq,Izz
  Bus Creator : BusCreator  Inputs=2
  Constant : Constant  Value=Imzz
  Constant1 : Constant  Value=I0
  Divide : Product  Inputs=*/
  Gain : Gain  Gain=1/L
  Gain1 : Gain  Gain=Km
  Gain3 : Gain  Gain=Kemf
  Gain4 : Gain  Gain=Ra
  Gain5 : Gain  Gain=1/(2*pi)
  Gain6 : Gain  Gain=60
  Integrator : Integrator
  Integrator1 : Integrator
  Multiply : Product
  Multiply1 : Product
  Terminator : Terminator
  Terminator1 : Terminator
  Out1 : Outport
  wires:
  Constant1/1 -> Add3/2
  Add3/1 -> Gain1/1  "Iav"
  [Tq] -> Add1/2
  Bus Creator/1 -> Out1/1
  Gain6/1 -> Bus Creator/2  "RPM"
  Gain5/1 -> Gain6/1  "RPS"
  Multiply1/1 -> Terminator1/1  "Pwout"
  Multiply/1 -> Terminator/1  "Pwin"
  [J] -> Divide/2
  Add2/1 -> [J]
  Constant/1 -> Add2/2
  Bus Selector/3 -> Add2/1  "<Izz>"
  Bus Selector/2 -> [Tq]  "<Tq>"
  Gain4/1 -> Add/3
  Gain3/1 -> Add/2  "Ea"
  Divide/1 -> Integrator1/1
  Add1/1 -> Divide/1
  Integrator1/1 -> Gain5/1, Gain3/1, Multiply1/2  "w"
  Gain1/1 -> Add1/1, Multiply1/1  "Te"
  Integrator/1 -> Gain4/1, Bus Creator/1, Multiply/2, Add3/1  "Im"
  Gain/1 -> Integrator/1
  Add/1 -> Gain/1
  Bus Selector/1 -> Add/1, Multiply/1  "<Um>"
  In1/1 -> Bus Selector/1

== system test_bu01_2018b/bu01_model/动力系统模型/Motor1_TM_P/TM1654P /螺旋桨模型/不做坐标转换 ==
  F_M : Inport
  Azb : Inport  Port=2
  Action Port : ActionPort  ActionType=then
  Bus Selector1 : BusSelector  OutputSignals=Fxp,Fyp,Fzp,Mxp,Myp,Mzp
  Bus Creator : BusCreator  Inputs=2
  Gain : Gain  Gain=Fratio
  Gain1 : Gain  Gain=Mratio
  Matrix Multiply : Product
  Matrix Multiply1 : Product
  Mux : Mux  Inputs=3
  Mux1 : Mux  Inputs=3
  Out1 : Outport
  wires:
  Bus Selector1/5 -> Mux1/2  "<Myp>"
  Bus Selector1/1 -> Mux/1  "<Fxp>"
  Mux/1 -> Matrix Multiply/2  "F"
  Bus Selector1/4 -> Mux1/1  "<Mxp>"
  Bus Selector1/2 -> Mux/2  "<Fyp>"
  F_M/1 -> Bus Selector1/1
  Mux1/1 -> Matrix Multiply1/2  "M"
  Bus Selector1/6 -> Mux1/3  "<Mzp>"
  Bus Selector1/3 -> Mux/3  "<Fzp>"
  Azb/1 -> Matrix Multiply1/1, Matrix Multiply/1
  Bus Creator/1 -> Out1/1
  Matrix Multiply/1 -> Gain/1
  Gain/1 -> Bus Creator/1  "Fb"
  Matrix Multiply1/1 -> Gain1/1
  Gain1/1 -> Bus Creator/2  "Mb"

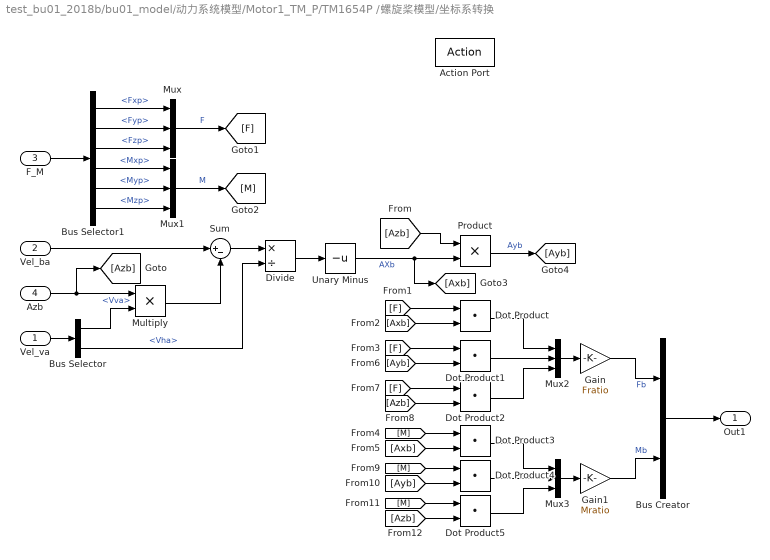
== system test_bu01_2018b/bu01_model/动力系统模型/Motor1_TM_P/TM1654P /螺旋桨模型/坐标系转换 ==
  Vel_va : Inport
  Vel_ba : Inport  Port=2
  F_M : Inport  Port=3
  Azb : Inport  Port=4
  Action Port : ActionPort  ActionType=else
  Bus Selector : BusSelector  OutputSignals=Vva,Vha
  Bus Selector1 : BusSelector  OutputSignals=Fxp,Fyp,Fzp,Mxp,Myp,Mzp
  Bus Creator : BusCreator  Inputs=2
  Divide : Product  Inputs=*/
  Dot Product{,1..5} (6 alike) : DotProduct  InputSameDT=on  OutDataTypeStr=Inherit: Inherit via internal rule
  Gain : Gain  Gain=Fratio
  Gain1 : Gain  Gain=Mratio
  Multiply : Product
  Mux{,1..3} (4 alike) : Mux  Inputs=3
  Product : Product
  Sum : Sum  Inputs=|+-
  Unary Minus : UnaryMinus
  Out1 : Outport
  wires:
  Azb/1 -> [Azb], Multiply/1
  Vel_va/1 -> Bus Selector/1
  Bus Selector/1 -> Multiply/2  "<Vva>"
  Bus Selector/2 -> Divide/2  "<Vha>"
  Vel_ba/1 -> Sum/1
  Multiply/1 -> Sum/2
  Sum/1 -> Divide/1
  Divide/1 -> Unary Minus/1
  Unary Minus/1 -> [Axb], Product/2  "AXb"
  [Azb] -> Product/1
  Product/1 -> [Ayb]  "Ayb"
  F_M/1 -> Bus Selector1/1
  Bus Selector1/1 -> Mux/1  "<Fxp>"
  Bus Selector1/3 -> Mux/3  "<Fzp>"
  Bus Selector1/2 -> Mux/2  "<Fyp>"
  Mux/1 -> [F]  "F"
  Bus Selector1/4 -> Mux1/1  "<Mxp>"
  Bus Selector1/5 -> Mux1/2  "<Myp>"
  Bus Selector1/6 -> Mux1/3  "<Mzp>"
  Mux1/1 -> [M]  "M"
  Dot Product/1 -> Mux2/1
  [M] -> Dot Product3/1
  [Axb] -> Dot Product3/2
  Dot Product3/1 -> Mux3/1
  [F] -> Dot Product/1
  [Axb] -> Dot Product/2
  [Ayb] -> Dot Product1/2
  Dot Product1/1 -> Mux2/2
  [F] -> Dot Product1/1
  [Azb] -> Dot Product2/2
  Dot Product2/1 -> Mux2/3
  [F] -> Dot Product2/1
  Mux2/1 -> Gain/1
  Dot Product4/1 -> Mux3/2
  [M] -> Dot Product4/1
  [Ayb] -> Dot Product4/2
  Dot Product5/1 -> Mux3/3
  [M] -> Dot Product5/1
  [Azb] -> Dot Product5/2
  Mux3/1 -> Gain1/1
  Gain1/1 -> Bus Creator/2  "Mb"
  Gain/1 -> Bus Creator/1  "Fb"
  Bus Creator/1 -> Out1/1

== system test_bu01_2018b/bu01_model/动力系统模型/Motor1_TM_P/TM1654P /螺旋桨模型/螺旋桨气动 ==
  V : Inport
  Ns : Inport  Port=2
  density : Inport  Port=3
  Abs : Abs
  Bus Selector : BusSelector  OutputSignals=Vva,Vha
  Bus Selector1 : BusSelector  OutputSignals=Mzp
  Bus Creator : BusCreator  Inputs=2
  Bus Creator1 : BusCreator  Inputs=6
  Constant : Constant  Value=D
  Constant1 : Constant  Value=D
  Constant2 : Constant  Value=4
  Constant3 : Constant  Value=[1;1; 1; D; D; D]
  Demux : Demux  Outputs=6
  Divide : Product  Inputs=*/
  Divide1 : Product  Inputs=*/
  Gain : Gain  Gain=Mratio
  Gain1 : Gain  Gain=2*pi
  Multiply : Product
  Multiply1 : Product  Inputs=4
  Multiply2 : Product
  Multiply3 : Product
  Ns1 : InportShadow  Port=2
  Ns2 : InportShadow  Port=2
  Square : Math  Operator=square  SaturateOnIntegerOverflow=on
  Square1 : Math  Operator=pow  OutputSignalType=real  SaturateOnIntegerOverflow=on
  Terminator : Terminator
  Unary Minus : UnaryMinus
  计算螺旋桨气动系数 : Subsystem
  F_M : Outport
  T_q : Outport  Port=2
  wires:
  V/1 -> Bus Selector/1
  Ns/1 -> Multiply/1
  Constant/1 -> Multiply/2
  Multiply/1 -> Divide1/2, Divide/2
  Bus Selector/2 -> Divide/1  "<Vha>"
  Divide/1 -> Bus Creator/2  "Miu"
  Bus Selector/1 -> Unary Minus/1  "<Vva>"
  Unary Minus/1 -> Divide1/1
  Divide1/1 -> Bus Creator/1  "Lumda"
  Bus Creator/1 -> 计算螺旋桨气动系数/1(In1)
  Ns1/1 -> Square/1
  Constant1/1 -> Square1/1
  Constant2/1 -> Square1/2
  Square/1 -> Multiply1/2
  Square1/1 -> Multiply1/3
  Constant3/1 -> Multiply2/1
  Multiply2/1 -> Demux/1
  Demux/1 -> Bus Creator1/1  "Fxp"
  Demux/2 -> Bus Creator1/2  "Fyp"
  Demux/3 -> Bus Creator1/3  "Fzp"
  Demux/4 -> Bus Creator1/4  "Mxp"
  Demux/5 -> Bus Creator1/5  "Myp"
  Demux/6 -> Bus Creator1/6  "Mzp"
  Bus Creator1/1 -> F_M/1, Bus Selector1/1
  Bus Selector1/1 -> Abs/1  "<Mzp>"
  Abs/1 -> Gain/1
  Gain/1 -> T_q/1, Multiply3/1  "Tq"
  Ns2/1 -> Multiply3/2
  Multiply3/1 -> Gain1/1
  Gain1/1 -> Terminator/1  "power"
  density/1 -> Multiply1/4
  计算螺旋桨气动系数/1(Out1) -> Multiply1/1
  Multiply1/1 -> Multiply2/2

== system test_bu01_2018b/bu01_model/动力系统模型/Motor2_TM_N/TM1654N /螺旋桨模型/不做坐标转换 ==
  F_M : Inport
  Azb : Inport  Port=2
  Action Port : ActionPort  ActionType=then
  Bus Selector1 : BusSelector  OutputSignals=Fxp,Fyp,Fzp,Mxp,Myp,Mzp
  Bus Creator : BusCreator  Inputs=2
  Gain : Gain  Gain=Fratio
  Gain1 : Gain  Gain=Mratio
  Matrix Multiply : Product
  Matrix Multiply1 : Product
  Mux : Mux  Inputs=3
  Mux1 : Mux  Inputs=3
  Out1 : Outport
  wires:
  Bus Selector1/5 -> Mux1/2  "<Myp>"
  Bus Selector1/1 -> Mux/1  "<Fxp>"
  Mux/1 -> Matrix Multiply/2  "F"
  Bus Selector1/4 -> Mux1/1  "<Mxp>"
  Bus Selector1/2 -> Mux/2  "<Fyp>"
  F_M/1 -> Bus Selector1/1
  Mux1/1 -> Matrix Multiply1/2  "M"
  Bus Selector1/6 -> Mux1/3  "<Mzp>"
  Bus Selector1/3 -> Mux/3  "<Fzp>"
  Azb/1 -> Matrix Multiply1/1, Matrix Multiply/1
  Bus Creator/1 -> Out1/1
  Matrix Multiply/1 -> Gain/1
  Gain/1 -> Bus Creator/1  "Fb"
  Matrix Multiply1/1 -> Gain1/1
  Gain1/1 -> Bus Creator/2  "Mb"

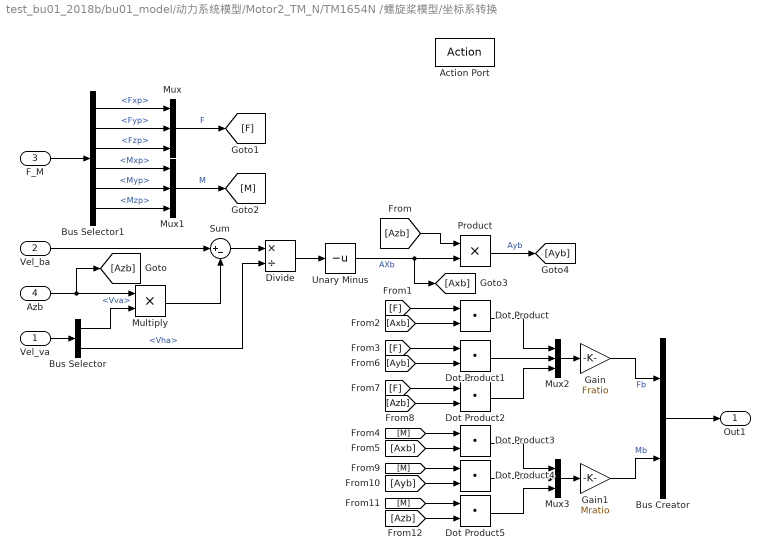
== system test_bu01_2018b/bu01_model/动力系统模型/Motor2_TM_N/TM1654N /螺旋桨模型/坐标系转换 ==
  Vel_va : Inport
  Vel_ba : Inport  Port=2
  F_M : Inport  Port=3
  Azb : Inport  Port=4
  Action Port : ActionPort  ActionType=else
  Bus Selector : BusSelector  OutputSignals=Vva,Vha
  Bus Selector1 : BusSelector  OutputSignals=Fxp,Fyp,Fzp,Mxp,Myp,Mzp
  Bus Creator : BusCreator  Inputs=2
  Divide : Product  Inputs=*/
  Dot Product{,1..5} (6 alike) : DotProduct  InputSameDT=on  OutDataTypeStr=Inherit: Inherit via internal rule
  Gain : Gain  Gain=Fratio
  Gain1 : Gain  Gain=Mratio
  Multiply : Product
  Mux{,1..3} (4 alike) : Mux  Inputs=3
  Product : Product
  Sum : Sum  Inputs=|+-
  Unary Minus : UnaryMinus
  Out1 : Outport
  wires:
  Azb/1 -> [Azb], Multiply/1
  Vel_va/1 -> Bus Selector/1
  Bus Selector/1 -> Multiply/2  "<Vva>"
  Bus Selector/2 -> Divide/2  "<Vha>"
  Vel_ba/1 -> Sum/1
  Multiply/1 -> Sum/2
  Sum/1 -> Divide/1
  Divide/1 -> Unary Minus/1
  Unary Minus/1 -> [Axb], Product/2  "AXb"
  [Azb] -> Product/1
  Product/1 -> [Ayb]  "Ayb"
  F_M/1 -> Bus Selector1/1
  Bus Selector1/1 -> Mux/1  "<Fxp>"
  Bus Selector1/3 -> Mux/3  "<Fzp>"
  Bus Selector1/2 -> Mux/2  "<Fyp>"
  Mux/1 -> [F]  "F"
  Bus Selector1/4 -> Mux1/1  "<Mxp>"
  Bus Selector1/5 -> Mux1/2  "<Myp>"
  Bus Selector1/6 -> Mux1/3  "<Mzp>"
  Mux1/1 -> [M]  "M"
  Dot Product/1 -> Mux2/1
  [M] -> Dot Product3/1
  [Axb] -> Dot Product3/2
  Dot Product3/1 -> Mux3/1
  [F] -> Dot Product/1
  [Axb] -> Dot Product/2
  [Ayb] -> Dot Product1/2
  Dot Product1/1 -> Mux2/2
  [F] -> Dot Product1/1
  [Azb] -> Dot Product2/2
  Dot Product2/1 -> Mux2/3
  [F] -> Dot Product2/1
  Mux2/1 -> Gain/1
  Dot Product4/1 -> Mux3/2
  [M] -> Dot Product4/1
  [Ayb] -> Dot Product4/2
  Dot Product5/1 -> Mux3/3
  [M] -> Dot Product5/1
  [Azb] -> Dot Product5/2
  Mux3/1 -> Gain1/1
  Gain1/1 -> Bus Creator/2  "Mb"
  Gain/1 -> Bus Creator/1  "Fb"
  Bus Creator/1 -> Out1/1

== system test_bu01_2018b/bu01_model/动力系统模型/Motor2_TM_N/TM1654N /螺旋桨模型/螺旋桨气动 ==
  V : Inport
  Ns : Inport  Port=2
  density : Inport  Port=3
  Abs : Abs
  Bus Selector : BusSelector  OutputSignals=Vva,Vha
  Bus Selector1 : BusSelector  OutputSignals=Mzp
  Bus Creator : BusCreator  Inputs=2
  Bus Creator1 : BusCreator  Inputs=6
  Constant : Constant  Value=D
  Constant1 : Constant  Value=D
  Constant2 : Constant  Value=4
  Constant3 : Constant  Value=[1;-1; 1; -D; D; -D]
  Demux : Demux  Outputs=6
  Divide : Product  Inputs=*/
  Divide1 : Product  Inputs=*/
  Gain : Gain  Gain=Mratio
  Gain1 : Gain  Gain=2*pi
  Multiply : Product
  Multiply1 : Product  Inputs=4
  Multiply2 : Product
  Multiply3 : Product
  Ns1 : InportShadow  Port=2
  Ns2 : InportShadow  Port=2
  Square : Math  Operator=square  SaturateOnIntegerOverflow=on
  Square1 : Math  Operator=pow  OutputSignalType=real  SaturateOnIntegerOverflow=on
  Terminator : Terminator
  Unary Minus : UnaryMinus
  计算螺旋桨气动系数 : Subsystem
  F_M : Outport
  T_q : Outport  Port=2
  wires:
  V/1 -> Bus Selector/1
  Ns/1 -> Multiply/1
  Constant/1 -> Multiply/2
  Multiply/1 -> Divide1/2, Divide/2
  Bus Selector/2 -> Divide/1  "<Vha>"
  Divide/1 -> Bus Creator/2  "Miu"
  Bus Selector/1 -> Unary Minus/1  "<Vva>"
  Unary Minus/1 -> Divide1/1
  Divide1/1 -> Bus Creator/1  "Lumda"
  Bus Creator/1 -> 计算螺旋桨气动系数/1(In1)
  Ns1/1 -> Square/1
  Constant1/1 -> Square1/1
  Constant2/1 -> Square1/2
  Square/1 -> Multiply1/2
  Square1/1 -> Multiply1/3
  Constant3/1 -> Multiply2/1
  Multiply2/1 -> Demux/1
  Demux/1 -> Bus Creator1/1  "Fxp"
  Demux/2 -> Bus Creator1/2  "Fyp"
  Demux/3 -> Bus Creator1/3  "Fzp"
  Demux/4 -> Bus Creator1/4  "Mxp"
  Demux/5 -> Bus Creator1/5  "Myp"
  Demux/6 -> Bus Creator1/6  "Mzp"
  Bus Creator1/1 -> F_M/1, Bus Selector1/1
  Bus Selector1/1 -> Abs/1  "<Mzp>"
  Abs/1 -> Gain/1
  Gain/1 -> T_q/1, Multiply3/1  "Tq"
  Ns2/1 -> Multiply3/2
  Multiply3/1 -> Gain1/1
  Gain1/1 -> Terminator/1  "power"
  density/1 -> Multiply1/4
  计算螺旋桨气动系数/1(Out1) -> Multiply1/1
  Multiply1/1 -> Multiply2/2

== system test_bu01_2018b/bu01_model/动力系统模型/Motor3_TM_P/TM1654P /螺旋桨模型/不做坐标转换 ==
  F_M : Inport
  Azb : Inport  Port=2
  Action Port : ActionPort  ActionType=then
  Bus Selector1 : BusSelector  OutputSignals=Fxp,Fyp,Fzp,Mxp,Myp,Mzp
  Bus Creator : BusCreator  Inputs=2
  Gain : Gain  Gain=Fratio
  Gain1 : Gain  Gain=Mratio
  Matrix Multiply : Product
  Matrix Multiply1 : Product
  Mux : Mux  Inputs=3
  Mux1 : Mux  Inputs=3
  Out1 : Outport
  wires:
  Bus Selector1/5 -> Mux1/2  "<Myp>"
  Bus Selector1/1 -> Mux/1  "<Fxp>"
  Mux/1 -> Matrix Multiply/2  "F"
  Bus Selector1/4 -> Mux1/1  "<Mxp>"
  Bus Selector1/2 -> Mux/2  "<Fyp>"
  F_M/1 -> Bus Selector1/1
  Mux1/1 -> Matrix Multiply1/2  "M"
  Bus Selector1/6 -> Mux1/3  "<Mzp>"
  Bus Selector1/3 -> Mux/3  "<Fzp>"
  Azb/1 -> Matrix Multiply1/1, Matrix Multiply/1
  Bus Creator/1 -> Out1/1
  Matrix Multiply/1 -> Gain/1
  Gain/1 -> Bus Creator/1  "Fb"
  Matrix Multiply1/1 -> Gain1/1
  Gain1/1 -> Bus Creator/2  "Mb"

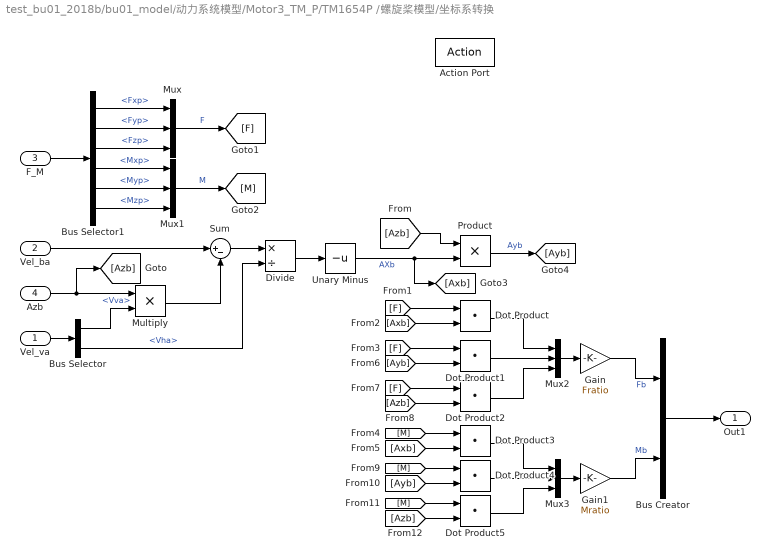
== system test_bu01_2018b/bu01_model/动力系统模型/Motor3_TM_P/TM1654P /螺旋桨模型/坐标系转换 ==
  Vel_va : Inport
  Vel_ba : Inport  Port=2
  F_M : Inport  Port=3
  Azb : Inport  Port=4
  Action Port : ActionPort  ActionType=else
  Bus Selector : BusSelector  OutputSignals=Vva,Vha
  Bus Selector1 : BusSelector  OutputSignals=Fxp,Fyp,Fzp,Mxp,Myp,Mzp
  Bus Creator : BusCreator  Inputs=2
  Divide : Product  Inputs=*/
  Dot Product{,1..5} (6 alike) : DotProduct  InputSameDT=on  OutDataTypeStr=Inherit: Inherit via internal rule
  Gain : Gain  Gain=Fratio
  Gain1 : Gain  Gain=Mratio
  Multiply : Product
  Mux{,1..3} (4 alike) : Mux  Inputs=3
  Product : Product
  Sum : Sum  Inputs=|+-
  Unary Minus : UnaryMinus
  Out1 : Outport
  wires:
  Azb/1 -> [Azb], Multiply/1
  Vel_va/1 -> Bus Selector/1
  Bus Selector/1 -> Multiply/2  "<Vva>"
  Bus Selector/2 -> Divide/2  "<Vha>"
  Vel_ba/1 -> Sum/1
  Multiply/1 -> Sum/2
  Sum/1 -> Divide/1
  Divide/1 -> Unary Minus/1
  Unary Minus/1 -> [Axb], Product/2  "AXb"
  [Azb] -> Product/1
  Product/1 -> [Ayb]  "Ayb"
  F_M/1 -> Bus Selector1/1
  Bus Selector1/1 -> Mux/1  "<Fxp>"
  Bus Selector1/3 -> Mux/3  "<Fzp>"
  Bus Selector1/2 -> Mux/2  "<Fyp>"
  Mux/1 -> [F]  "F"
  Bus Selector1/4 -> Mux1/1  "<Mxp>"
  Bus Selector1/5 -> Mux1/2  "<Myp>"
  Bus Selector1/6 -> Mux1/3  "<Mzp>"
  Mux1/1 -> [M]  "M"
  Dot Product/1 -> Mux2/1
  [M] -> Dot Product3/1
  [Axb] -> Dot Product3/2
  Dot Product3/1 -> Mux3/1
  [F] -> Dot Product/1
  [Axb] -> Dot Product/2
  [Ayb] -> Dot Product1/2
  Dot Product1/1 -> Mux2/2
  [F] -> Dot Product1/1
  [Azb] -> Dot Product2/2
  Dot Product2/1 -> Mux2/3
  [F] -> Dot Product2/1
  Mux2/1 -> Gain/1
  Dot Product4/1 -> Mux3/2
  [M] -> Dot Product4/1
  [Ayb] -> Dot Product4/2
  Dot Product5/1 -> Mux3/3
  [M] -> Dot Product5/1
  [Azb] -> Dot Product5/2
  Mux3/1 -> Gain1/1
  Gain1/1 -> Bus Creator/2  "Mb"
  Gain/1 -> Bus Creator/1  "Fb"
  Bus Creator/1 -> Out1/1

== system test_bu01_2018b/bu01_model/动力系统模型/Motor3_TM_P/TM1654P /螺旋桨模型/螺旋桨气动 ==
  V : Inport
  Ns : Inport  Port=2
  density : Inport  Port=3
  Abs : Abs
  Bus Selector : BusSelector  OutputSignals=Vva,Vha
  Bus Selector1 : BusSelector  OutputSignals=Mzp
  Bus Creator : BusCreator  Inputs=2
  Bus Creator1 : BusCreator  Inputs=6
  Constant : Constant  Value=D
  Constant1 : Constant  Value=D
  Constant2 : Constant  Value=4
  Constant3 : Constant  Value=[1;1; 1; D; D; D]
  Demux : Demux  Outputs=6
  Divide : Product  Inputs=*/
  Divide1 : Product  Inputs=*/
  Gain : Gain  Gain=Mratio
  Gain1 : Gain  Gain=2*pi
  Multiply : Product
  Multiply1 : Product  Inputs=4
  Multiply2 : Product
  Multiply3 : Product
  Ns1 : InportShadow  Port=2
  Ns2 : InportShadow  Port=2
  Square : Math  Operator=square  SaturateOnIntegerOverflow=on
  Square1 : Math  Operator=pow  OutputSignalType=real  SaturateOnIntegerOverflow=on
  Terminator : Terminator
  Unary Minus : UnaryMinus
  计算螺旋桨气动系数 : Subsystem
  F_M : Outport
  T_q : Outport  Port=2
  wires:
  V/1 -> Bus Selector/1
  Ns/1 -> Multiply/1
  Constant/1 -> Multiply/2
  Multiply/1 -> Divide1/2, Divide/2
  Bus Selector/2 -> Divide/1  "<Vha>"
  Divide/1 -> Bus Creator/2  "Miu"
  Bus Selector/1 -> Unary Minus/1  "<Vva>"
  Unary Minus/1 -> Divide1/1
  Divide1/1 -> Bus Creator/1  "Lumda"
  Bus Creator/1 -> 计算螺旋桨气动系数/1(In1)
  Ns1/1 -> Square/1
  Constant1/1 -> Square1/1
  Constant2/1 -> Square1/2
  Square/1 -> Multiply1/2
  Square1/1 -> Multiply1/3
  Constant3/1 -> Multiply2/1
  Multiply2/1 -> Demux/1
  Demux/1 -> Bus Creator1/1  "Fxp"
  Demux/2 -> Bus Creator1/2  "Fyp"
  Demux/3 -> Bus Creator1/3  "Fzp"
  Demux/4 -> Bus Creator1/4  "Mxp"
  Demux/5 -> Bus Creator1/5  "Myp"
  Demux/6 -> Bus Creator1/6  "Mzp"
  Bus Creator1/1 -> F_M/1, Bus Selector1/1
  Bus Selector1/1 -> Abs/1  "<Mzp>"
  Abs/1 -> Gain/1
  Gain/1 -> T_q/1, Multiply3/1  "Tq"
  Ns2/1 -> Multiply3/2
  Multiply3/1 -> Gain1/1
  Gain1/1 -> Terminator/1  "power"
  density/1 -> Multiply1/4
  计算螺旋桨气动系数/1(Out1) -> Multiply1/1
  Multiply1/1 -> Multiply2/2
